simulink model "chop1q_ifb_simulink_r13"  (Simulink 5.1)
settings: Solver=ode5  StartTime=0.0  StopTime=1.5e-3  FixedStep=2e-6  RelTol=1e-3
settings Model: LastModifiedBy=user  LimitDataPoints=off  ProdHWDeviceType=Microprocessor

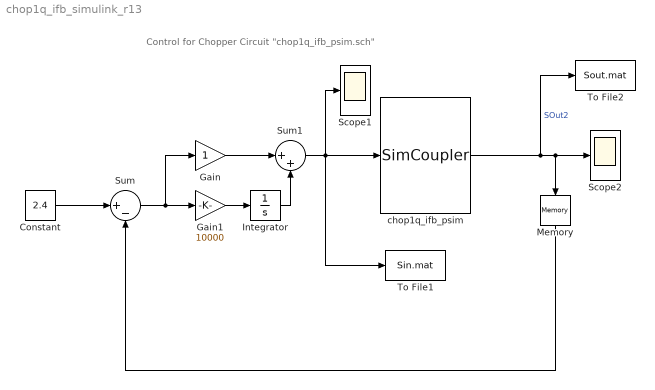
== system chop1q_ifb_simulink_r13 ==
  note: Control for Chopper Circuit "chop1q_ifb_psim.sch"
  Constant : Constant  Value=2.4
  Gain : Gain  SaturateOnIntegerOverflow=on
  Gain1 : Gain  Gain=10000  SaturateOnIntegerOverflow=on
  Integrator : Integrator
  Memory : Memory  Orientation=down
  Scope1 : Scope
      settings: TimeRange=0.04  YMin=-40  YMax=60
  Scope2 : Scope
      settings: TimeRange=0.04  YMin=-40  YMax=60
  Sum : Sum  Inputs=|+-  SaturateOnIntegerOverflow=on  InputSameDT=on
  Sum1 : Sum  Inputs=|++  SaturateOnIntegerOverflow=on  InputSameDT=on
  To File1 : ToFile  Filename=Sin.mat
  To File2 : ToFile  Filename=Sout.mat
  chop1q_ifb_psim : S-Function  FunctionName=SimCoupler  Parameters='C:\PSIM\examples\SimCoupler\chop1q_ifb_psim.sch'  mask(SimCoupler){Netlist_File=C:\PSIM6.1\examples\simcoupler\chop1q_ifb_psim.cct}
      mask prompts: Netlist_File "Model Netlist File"
      mask init:
      | c=[0:10:360]*pi/180;
      | x1=cos(c)*30; y1=sin(c)*30+20;
      | x2=cos(c)*30;y2=sin(c)*30-20;
      settings: OpenFcn=PSimDialog('PSimFileEdt','Value','Parameters');
      mask Display:
      | plot(-60,-60,60,60,x1,y1,x2,y2)
      | port_label('input', 1, 'Vm')
      | port_label('output', 1, 'iL')
  wires:
  Constant/1 -> Sum/1
  Sum/1 -> Gain/1, Gain1/1
  Gain/1 -> Sum1/1
  Gain1/1 -> Integrator/1
  Integrator/1 -> Sum1/2
  Sum1/1 -> chop1q_ifb_psim/1, Scope1/1, To File1/1
  chop1q_ifb_psim/1 -> Scope2/1, Memory/1, To File2/1  "SOut2"
  Memory/1 -> Sum/2
